simulink model "threestagesteam"  (R2024b)
settings: Solver=VariableStepAuto  StartTime=0.0  StopTime=30  RelTol=1e-3
settings Model: Creator=aspar  LastModifiedBy=aspar

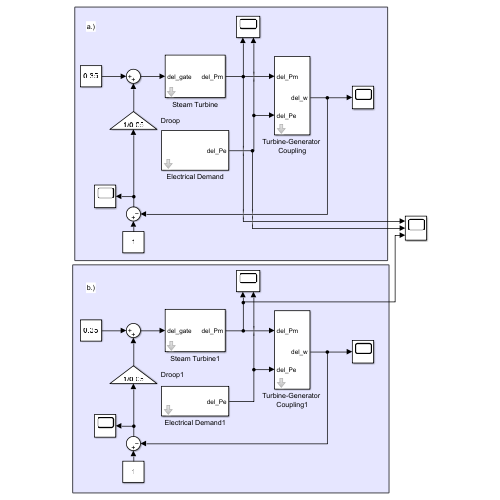
[thumbnail: Simulink's stored preview of the top-level diagram]
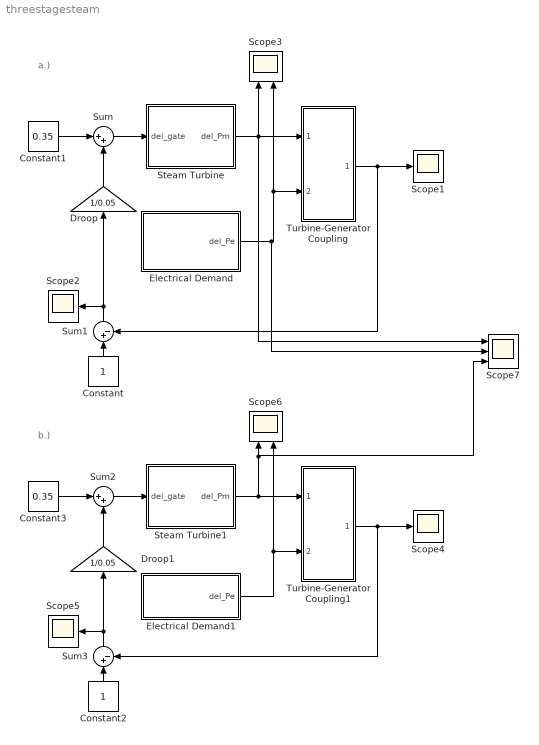
== system threestagesteam ==
  note: a.)
  note: b.)
  Constant : Constant
  Constant1 : Constant  Value=0.35
  Constant2 : Constant
  Constant3 : Constant  Value=0.35
  Droop : Gain  Gain=1/0.05
  Droop1 : Gain  Gain=1/0.05
  Electrical Demand : Subsystem  mask{initial_val=0.35}
  Electrical Demand1 : Subsystem  mask{initial_val=0.35}
  Scope{1..2,4..5} (4 alike) : Scope
  Scope3 : Scope  NumInputPorts=2
  Scope6 : Scope  NumInputPorts=2
  Scope7 : Scope  NumInputPorts=3
  Steam Turbine : Subsystem  mask{ini=0.35}
  Steam Turbine1 : Subsystem  mask{ini=0.35}
  Sum : Sum  Inputs=|++
  Sum1 : Sum  Inputs=|+-
  Sum2 : Sum  Inputs=|++
  Sum3 : Sum  Inputs=|+-
  Turbine-Generator Coupling : Subsystem  mask{H=1.2, initi=1}
  Turbine-Generator Coupling1 : Subsystem  mask{H=1.2, initi=1}
  wires:
  Sum/1 -> Steam Turbine/1(del_gate)
  Turbine-Generator Coupling/1(del_w) -> Sum1/2, Scope1/1
  Constant/1 -> Sum1/1
  Constant1/1 -> Sum/1
  Droop/1 -> Sum/2
  Sum1/1 -> Droop/1, Scope2/1
  Steam Turbine/1(del_Pm) -> Scope3/1, Scope7/1, Turbine-Generator Coupling/1(del_Pm)
  Electrical Demand/1(del_Pe) -> Scope7/2, Scope3/2, Turbine-Generator Coupling/2(del_Pe)
  Electrical Demand1/1(del_Pe) -> Scope6/2, Turbine-Generator Coupling1/2(del_Pe)
  Sum2/1 -> Steam Turbine1/1(del_gate)
  Constant3/1 -> Sum2/1
  Steam Turbine1/1(del_Pm) -> Turbine-Generator Coupling1/1(del_Pm), Scope7/3, Scope6/1
  Sum3/1 -> Droop1/1, Scope5/1
  Constant2/1 -> Sum3/1
  Turbine-Generator Coupling1/1(del_w) -> Sum3/2, Scope4/1
  Droop1/1 -> Sum2/2

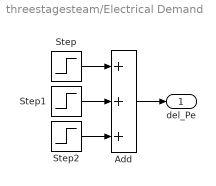
== system threestagesteam/Electrical Demand ==
  Add : Sum  Inputs=+++
  Step : Step  Time=5  Before=initial_val  After=0.6  SampleTime=0
  Step1 : Step  Time=15  After=-0.2  SampleTime=0
  Step2 : Step  Time=20  After=0.35  SampleTime=0
  del_Pe : Outport
  wires:
  Step1/1 -> Add/2
  Step2/1 -> Add/3
  Step/1 -> Add/1
  Add/1 -> del_Pe/1

== system threestagesteam/Electrical Demand1 ==
  Add : Sum  Inputs=+++
  Step : Step  Time=5  Before=initial_val  After=0.6  SampleTime=0
  Step1 : Step  Time=15  After=-0.2  SampleTime=0
  Step2 : Step  Time=20  After=0.35  SampleTime=0
  del_Pe : Outport
  wires:
  Step1/1 -> Add/2
  Step2/1 -> Add/3
  Step/1 -> Add/1
  Add/1 -> del_Pe/1

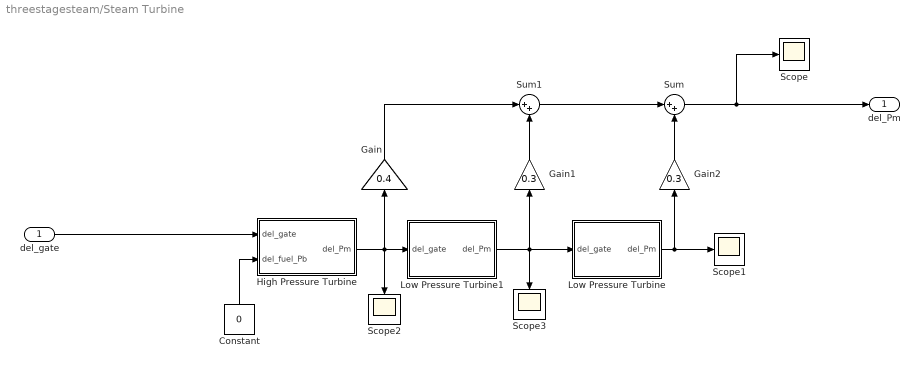
== system threestagesteam/Steam Turbine ==
  del_gate : Inport
  Constant : Constant  Value=0
  Gain : Gain  Gain=0.4
  Gain1 : Gain  Gain=0.3
  Gain2 : Gain  Gain=0.3
  High Pressure Turbine : Subsystem  mask{Th=0.3, init=ini}
  Low Pressure Turbine : Subsystem  mask{Tl=0.35, init=ini}
  Low Pressure Turbine1 : Subsystem  mask{Tl=0.4, init=ini}
  Scope{,1..3} (4 alike) : Scope
  Sum : Sum  Inputs=|++
  Sum1 : Sum  Inputs=|++
  del_Pm : Outport
  wires:
  Gain1/1 -> Sum1/2
  Gain/1 -> Sum1/1
  Constant/1 -> High Pressure Turbine/2(del_fuel_Pb)
  Sum1/1 -> Sum/1
  Low Pressure Turbine1/1(del_Pm) -> Scope3/1, Low Pressure Turbine/1(del_gate), Gain1/1
  Low Pressure Turbine/1(del_Pm) -> Scope1/1, Gain2/1
  Gain2/1 -> Sum/2
  High Pressure Turbine/1(del_Pm) -> Scope2/1, Low Pressure Turbine1/1(del_gate), Gain/1
  del_gate/1 -> High Pressure Turbine/1(del_gate)
  Sum/1 -> Scope/1, del_Pm/1

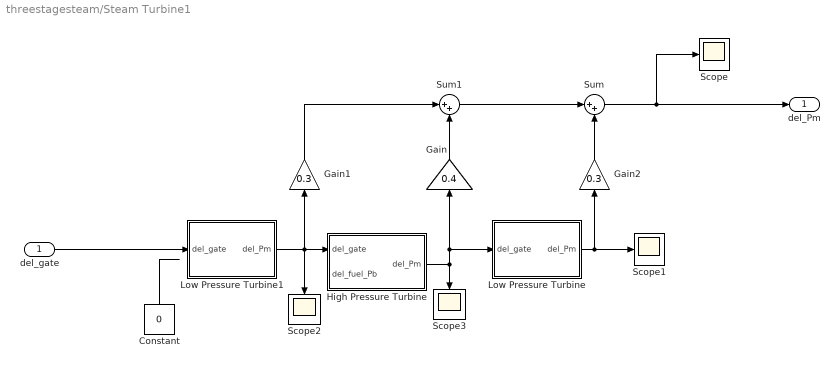
== system threestagesteam/Steam Turbine1 ==
  del_gate : Inport
  Constant : Constant  Value=0
  Gain : Gain  Gain=0.4
  Gain1 : Gain  Gain=0.3
  Gain2 : Gain  Gain=0.3
  High Pressure Turbine : Subsystem  mask{Th=0.3, init=ini}
  Low Pressure Turbine : Subsystem  mask{Tl=0.35, init=ini}
  Low Pressure Turbine1 : Subsystem  mask{Tl=0.4, init=ini}
  Scope{,1..3} (4 alike) : Scope
  Sum : Sum  Inputs=|++
  Sum1 : Sum  Inputs=|++
  del_Pm : Outport
  wires:
  Gain/1 -> Sum1/2
  Gain1/1 -> Sum1/1
  Constant/1 -> ?
  Sum1/1 -> Sum/1
  High Pressure Turbine/1(del_Pm) -> Gain/1, Low Pressure Turbine/1(del_gate), Scope3/1
  Low Pressure Turbine/1(del_Pm) -> Scope1/1, Gain2/1
  Gain2/1 -> Sum/2
  Low Pressure Turbine1/1(del_Pm) -> Gain1/1, High Pressure Turbine/1(del_gate), Scope2/1
  del_gate/1 -> Low Pressure Turbine1/1(del_gate)
  Sum/1 -> Scope/1, del_Pm/1

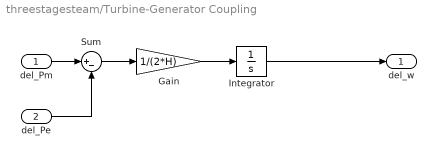
== system threestagesteam/Turbine-Generator Coupling ==
  del_Pm : Inport
  del_Pe : Inport  Port=2
  Gain : Gain  Gain=1/(2*H)
  Integrator : Integrator  InitialCondition=initi
  Sum : Sum  Inputs=|+-
  del_w : Outport
  wires:
  Gain/1 -> Integrator/1
  Integrator/1 -> del_w/1
  Sum/1 -> Gain/1
  del_Pm/1 -> Sum/1
  del_Pe/1 -> Sum/2

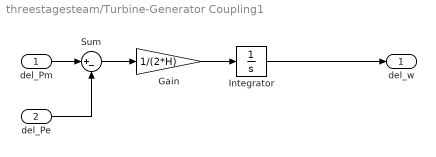
== system threestagesteam/Turbine-Generator Coupling1 ==
  del_Pm : Inport
  del_Pe : Inport  Port=2
  Gain : Gain  Gain=1/(2*H)
  Integrator : Integrator  InitialCondition=initi
  Sum : Sum  Inputs=|+-
  del_w : Outport
  wires:
  Gain/1 -> Integrator/1
  Integrator/1 -> del_w/1
  Sum/1 -> Gain/1
  del_Pm/1 -> Sum/1
  del_Pe/1 -> Sum/2

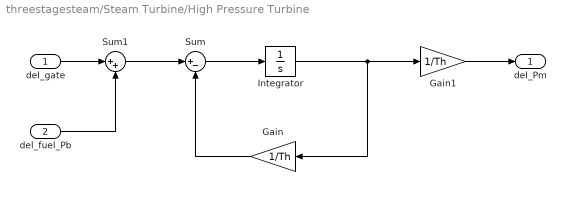
== system threestagesteam/Steam Turbine/High Pressure Turbine ==
  del_gate : Inport
  del_fuel_Pb : Inport  Port=2
  Gain : Gain  Gain=1/Th
  Gain1 : Gain  Gain=1/Th
  Integrator : Integrator  InitialCondition=Th*ini
  Sum : Sum  Inputs=|+-
  Sum1 : Sum  Inputs=|++
  del_Pm : Outport
  wires:
  Sum/1 -> Integrator/1
  Sum1/1 -> Sum/1
  Gain/1 -> Sum/2
  del_gate/1 -> Sum1/1
  Integrator/1 -> Gain/1, Gain1/1
  del_fuel_Pb/1 -> Sum1/2
  Gain1/1 -> del_Pm/1

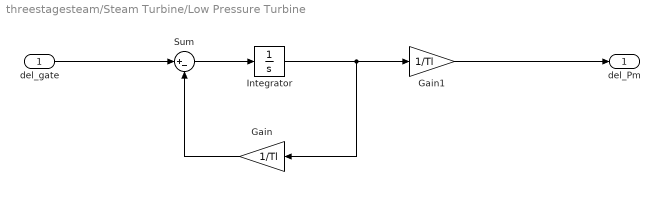
== system threestagesteam/Steam Turbine/Low Pressure Turbine ==
  del_gate : Inport
  Gain : Gain  Gain=1/Tl
  Gain1 : Gain  Gain=1/Tl
  Integrator : Integrator  InitialCondition=Tl*ini
  Sum : Sum  Inputs=|+-
  del_Pm : Outport
  wires:
  Sum/1 -> Integrator/1
  del_gate/1 -> Sum/1
  Gain/1 -> Sum/2
  Integrator/1 -> Gain/1, Gain1/1
  Gain1/1 -> del_Pm/1

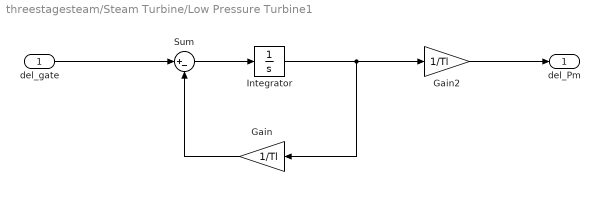
== system threestagesteam/Steam Turbine/Low Pressure Turbine1 ==
  del_gate : Inport
  Gain : Gain  Gain=1/Tl
  Gain2 : Gain  Gain=1/Tl
  Integrator : Integrator  InitialCondition=Tl*ini
  Sum : Sum  Inputs=|+-
  del_Pm : Outport
  wires:
  Sum/1 -> Integrator/1
  Integrator/1 -> Gain2/1, Gain/1
  del_gate/1 -> Sum/1
  Gain/1 -> Sum/2
  Gain2/1 -> del_Pm/1

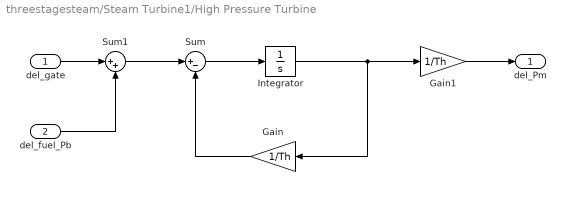
== system threestagesteam/Steam Turbine1/High Pressure Turbine ==
  del_gate : Inport
  del_fuel_Pb : Inport  Port=2
  Gain : Gain  Gain=1/Th
  Gain1 : Gain  Gain=1/Th
  Integrator : Integrator  InitialCondition=Th*ini
  Sum : Sum  Inputs=|+-
  Sum1 : Sum  Inputs=|++
  del_Pm : Outport
  wires:
  Sum/1 -> Integrator/1
  Sum1/1 -> Sum/1
  Gain/1 -> Sum/2
  del_gate/1 -> Sum1/1
  Integrator/1 -> Gain/1, Gain1/1
  del_fuel_Pb/1 -> Sum1/2
  Gain1/1 -> del_Pm/1

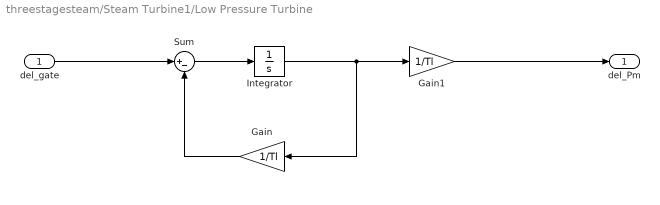
== system threestagesteam/Steam Turbine1/Low Pressure Turbine ==
  del_gate : Inport
  Gain : Gain  Gain=1/Tl
  Gain1 : Gain  Gain=1/Tl
  Integrator : Integrator  InitialCondition=Tl*ini
  Sum : Sum  Inputs=|+-
  del_Pm : Outport
  wires:
  Sum/1 -> Integrator/1
  del_gate/1 -> Sum/1
  Gain/1 -> Sum/2
  Integrator/1 -> Gain/1, Gain1/1
  Gain1/1 -> del_Pm/1

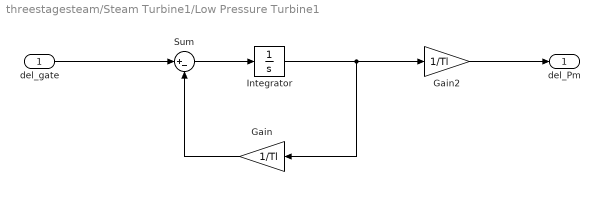
== system threestagesteam/Steam Turbine1/Low Pressure Turbine1 ==
  del_gate : Inport
  Gain : Gain  Gain=1/Tl
  Gain2 : Gain  Gain=1/Tl
  Integrator : Integrator  InitialCondition=Tl*ini
  Sum : Sum  Inputs=|+-
  del_Pm : Outport
  wires:
  Sum/1 -> Integrator/1
  Integrator/1 -> Gain2/1, Gain/1
  del_gate/1 -> Sum/1
  Gain/1 -> Sum/2
  Gain2/1 -> del_Pm/1
